simulink subsystem "ChargerThermalDummy"  (R2024b)
settings: Solver=VariableStepAuto  StartTime=0.0  StopTime=10.0  RelTol=1e-3
Description:
  | Charger with Thermal Model
  | 
  | ⚡ Main Features:
  | - Constant-current, constant-voltage (CC–CV) charging control
  | - Inputs: relay command, battery cell voltage, and charging status
  | - Controlled current source to HV bus for charging power
  | - Thermal representation of charger converter with heat generation
  | - Coupled to coolant jacket for thermal management
  | 
  | 📤 Outputs: Charging Current, HV Power, Converter Thermal States
  | 
  | 📌 Use Case: Study charging dynamics and thermal behavior of onboard charger
settings Model: Creator=saprasad  LastModifiedBy=jjha
settings RTWCC: GPUComputeCapability=3.5

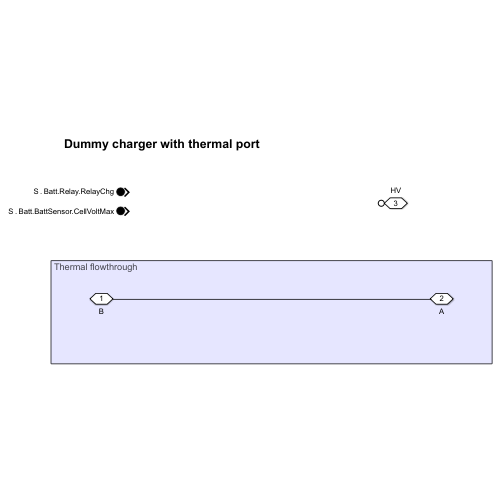
[thumbnail: Simulink's stored preview of the top-level diagram]
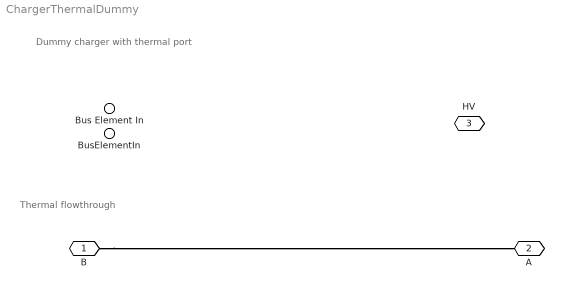
== system ChargerThermalDummy ==
  note: Dummy charger with thermal port
  note: Thermal flowthrough
  Bus Element In : Inport  PortName=S  Element=Batt.Relay.RelayChg
  BusElementIn : Inport  PortName=S  Element=Batt.BattSensor.CellVoltMax
  B : PMIOPort  Side=Left
  A : PMIOPort  Port=2  Side=Right
  HV : PMIOPort  Port=3  Side=Left
  connections:
  B/RConn1 -- A/RConn1
